simulink model "height_control"  (R2016b)
settings: Solver=VariableStepAuto  StartTime=0.0  StopTime=10.0  RelTol=1e-3
undefined symbols (not defined in the file): D, I, P
settings Model: Creator=Bryce  LastModifiedBy=Bryce

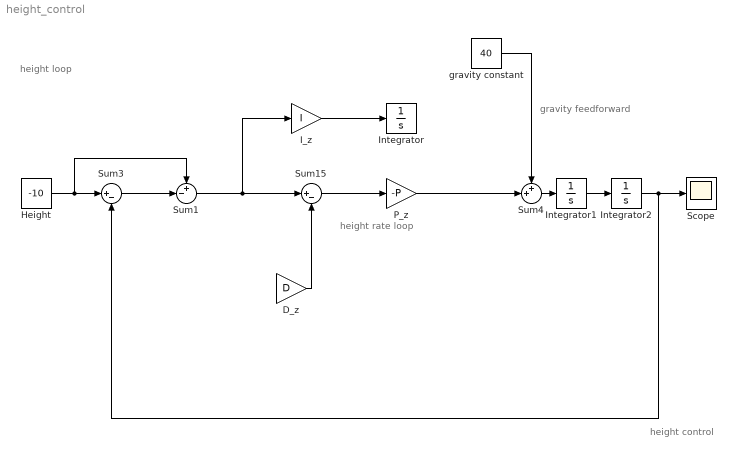
== system height_control ==
  note: height control
  note: gravity feedforward
  note: height rate
      | loop
  note: height
      | loop
  D_z : Gain  Gain=D
  Height : Constant  Value=-10  SampleTime=0
  I_z : Gain  Gain=I
  Integrator : Integrator
  Integrator1 : Integrator
  Integrator2 : Integrator
  P_z : Gain  Gain=-P
  Scope : Scope
  Sum1 : Sum  Inputs=+-|
  Sum15 : Sum  Inputs=|+-
  Sum3 : Sum  Inputs=|+-
  Sum4 : Sum  Inputs=++|
  "gravity constant " : Constant  Value=40  SampleTime=0
  wires:
  Sum15/1 -> P_z/1
  P_z/1 -> Sum4/2
  Height/1 -> Sum1/1, Sum3/1
  D_z/1 -> Sum15/2
  I_z/1 -> Integrator/1
  "gravity constant "/1 -> Sum4/1
  Integrator1/1 -> Integrator2/1
  Integrator2/1 -> Sum3/2, Scope/1
  Sum4/1 -> Integrator1/1
  Sum1/1 -> I_z/1, Sum15/1
  Sum3/1 -> Sum1/2
